simulink model "faulhaber_1524E006M485"  (R2019b)
settings: Solver=VariableStepAuto  StartTime=0.0  StopTime=40  MaxStep=.01  RelTol=1e-3
libraries: vrlib x2
settings Model: Creator=humms  LastModifiedBy=humms

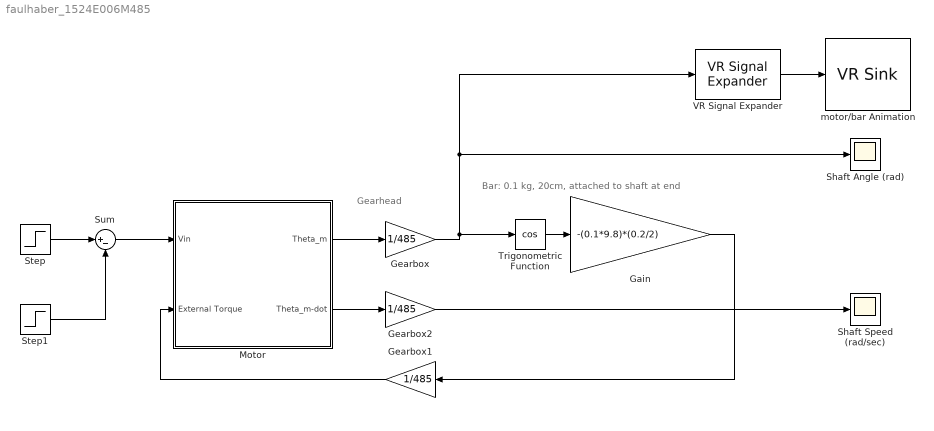
== system faulhaber_1524E006M485 ==
  note: Bar: 0.1 kg, 20cm, attached to shaft at end
  note: Gearhead
  Gain : Gain  Gain=-(0.1*9.8)*(0.2/2)
  Gearbox : Gain  Gain=1/485
  Gearbox1 : Gain  Gain=1/485
  Gearbox2 : Gain  Gain=1/485
  Motor : Subsystem
  Shaft Angle (rad) : Scope
  Shaft Speed (rad/sec) : Scope
  Step : Step  Time=5  After=5  SampleTime=0
  Step1 : Step  Time=20  After=5  SampleTime=0
  Sum : Sum  Inputs=|+-
  Trigonometric Function : Trigonometry  Operator=cos
  VR Signal Expander : vrlib/VR Signal Expander  outwidth=4  outidx=[4]
      settings: SourceProductName=Simulink
  motor/bar Animation : vrlib/VR Sink  InstantiateOnLoad=on  SampleTime=0.02  ViewEnable=on  RemoteChange=off  RemoteView=off  FieldsWritten=Bar.rotation.4.1.1.double  WorldFileName=rotating_bar.wrl  AutoView=off  VideoDimensions=[]  AllowVariableSize=off  FigureProperties="{'Position', 'Name', 'Viewpoint', 'CameraBound', 'CameraDirection', 'CameraPosition', 'CameraUpVector', 'ZoomFactor', 'Antialiasing', 'Headlight', 'Lighting', 'NavPanel', 'Sound', 'StatusBar', 'Stereo3D', 'Stereo3DCameraOffset', 'Stereo3DHIT', 'ToolBar', 'Textures', 'Transparency', 'Triad', 'Wireframe', 'NavZones', 'NavMode', 'NavSpeed', 'CaptureFileFormat', 'CaptureFileName', 'Record2DCompressMethod', 'Record2DCompressQuality', 'Record2D', 'Record2DFileName', 'Record2DFPS'; [1.0000000000000000e+00   9.3000000000000000e+01   5.7600000000000000e+02   3.5000000000000000e+02], '', 'Front View', 'on', [0.0000000000000000e+00   0.0000000000000000e+00  -1.0000000000000000e+00], [0.0000000000000000e+00   0.0000000000000000e+00   0.0000000000000000e+00], [0.0000000000000000e+00   1.0000000000000000e+00   0.0000000000000000e+00], [1.0000000000000000e+00], 'on', 'on', 'on', 'halfbar', 'on', 'on', 'off', [1.0000000149011612e-01], [0.0000000000000000e+00], 'on', 'on', 'on', 'none', 'off', 'off', 'fly', 'normal', 'tif', '%f_anim_%n.tif', 'auto', [7.5000000000000000e+01], 'off', '%f_anim_%n.avi', 'auto'}"
      settings: SourceProductName=Simulink
  wires:
  Motor/1(Theta_m) -> Gearbox/1
  Gearbox1/1 -> Motor/2(External Torque)
  Gain/1 -> Gearbox1/1
  Trigonometric Function/1 -> Gain/1
  Step/1 -> Sum/1
  Step1/1 -> Sum/2
  Sum/1 -> Motor/1(Vin)
  Motor/2(Theta_m-dot) -> Gearbox2/1
  Gearbox2/1 -> Shaft Speed (rad/sec)/1
  Gearbox/1 -> VR Signal Expander/1, Shaft Angle (rad)/1, Trigonometric Function/1
  VR Signal Expander/1 -> motor/bar Animation/1

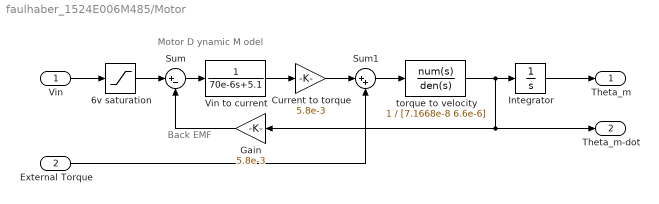
== system faulhaber_1524E006M485/Motor ==
  note: Back EMF
  note: Motor D ynamic M odel
  Vin : Inport
  External Torque : Inport  Port=2
  6v saturation : Saturate  UpperLimit=6  LowerLimit=-6
  Current to torque : Gain  Gain=5.8e-3
  Gain : Gain  Gain=5.8e-3
  Integrator : Integrator
  Sum : Sum  Inputs=|+-
  Sum1 : Sum  Inputs=|++
  Vin to current : TransferFcn  Denominator=[70e-6 5.1]
  torque to velocity : TransferFcn  Numerator=1  Denominator=[7.1668e-8 6.6e-6]
  Theta_m : Outport
  Theta_m-dot : Outport  Port=2
  wires:
  Sum/1 -> Vin to current/1
  Vin to current/1 -> Current to torque/1
  Integrator/1 -> Theta_m/1
  torque to velocity/1 -> Gain/1, Theta_m-dot/1, Integrator/1
  Gain/1 -> Sum/2
  Current to torque/1 -> Sum1/1
  External Torque/1 -> Sum1/2
  Sum1/1 -> torque to velocity/1
  Vin/1 -> 6v saturation/1
  6v saturation/1 -> Sum/1
